simulink model "ModeStEnCtrlCaller"  (R2018b)
settings: Solver=FixedStepDiscrete  StartTime=0.0  StopTime=10.0  FixedStep=0.01  RelTol=1e-3
undefined symbols (not defined in the file): MdXX_DoneChk_Cal, ModeStEnCtrl4s_Cal, ModeStEnCtrl6s7s_Cal, ModeStEnCtrl6s7sPreCondition_Cal
settings Model: Creator=sn2xws  LastModifiedBy=sn2xws
settings DataIOCC: SaveFormat=StructureWithTime
settings OptimizationCC: DefaultParameterBehavior=Inlined  EnhancedBackFolding=on  PassReuseOutputArgsAs=Individual arguments  ZeroExternalMemoryAtStartup=off  ZeroInternalMemoryAtStartup=off  OptimizeBlockOrder=speed  DifferentSizesBufferReuse=on  OptimizationCustomize=off
settings DebuggingCC: ParameterTunabilityLossMsg=error
settings SFSimCC: MATLABDynamicMemAlloc=off
settings RTWCC: SystemTargetFile=autosar.tlc  GenCodeOnly=on  TemplateMakefile=ert_default_tmf  Description=AUTOSAR  GenerateReport=on  IncludeHyperlinkInReport=on  LaunchReport=on  GenerateTraceInfo=on  GenerateTraceReport=on  GenerateTraceReportSl=on  GenerateTraceReportSf=on  GenerateTraceReportEml=on  GenerateCodeMetricsReport=on
settings CodeAppCC: ForceParamTrailComments=on  IgnoreCustomStorageClasses=off  OperatorAnnotations=on  SimulinkDataObjDesc=on  SFDataObjDesc=on  InsertBlockDesc=on
settings STFCustomTargetCC: TargetLangStandard=C99 (ISO)  MultiwordLength=256  ParMdlRefBuildCompliant=on  CompOptLevelCompliant=on  IncludeMdlTerminateFcn=off  CombineOutputUpdateFcns=on  SuppressErrorStatus=on  ERTCustomFileBanners=on  SupportNonFinite=off  SupportComplex=off  SupportContinuousTime=off  SupportNonInlinedSFcns=off  RemoveResetFunc=on  MATLABClassNameForMDSCustomization=Simulink.SoftwareTarget.ERTCustomization  AutosarCompliant=on  UseToolchainInfoCompliant=on  LookupTableObjectStructAxisOrder=2,1,3,4,...  LUTObjectStructOrderEvenSpacing=Size,Table,Breakpoints  SystemTargetFile=autosar.tlc
settings ERTTargetCC: TargetLangStandard=C99 (ISO)  ConcurrentExecutionCompliant=off  IncludeMdlTerminateFcn=off  SuppressErrorStatus=on  SupportNonFinite=off  SupportComplex=off  ModelStepFunctionPrototypeControlCompliant=off  CPPClassGenCompliant=off  AutosarCompliant=on  LookupTableObjectStructAxisOrder=2,1,3,4,...  LUTObjectStructOrderEvenSpacing=Size,Table,Breakpoints  InlinedParameterPlacement=NonHierarchical  ERTCustomFileTemplate=example_file_process.tlc  ERTFilePackagingFormat=Compact

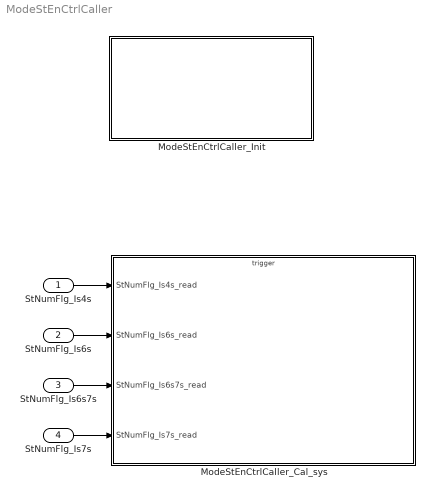
== system ModeStEnCtrlCaller ==
  StNumFlg_Is4s : Inport  OutDataTypeStr=boolean  PortDimensions=1
  StNumFlg_Is6s : Inport  Port=2  OutDataTypeStr=boolean  PortDimensions=1
  StNumFlg_Is6s7s : Inport  Port=3  OutDataTypeStr=boolean  PortDimensions=1
  StNumFlg_Is7s : Inport  Port=4  OutDataTypeStr=boolean  PortDimensions=1
  ModeStEnCtrlCaller_Cal_sys : Subsystem
  ModeStEnCtrlCaller_Init : Subsystem
  wires:
  StNumFlg_Is4s/1 -> ModeStEnCtrlCaller_Cal_sys/1(StNumFlg_Is4s_read)
  StNumFlg_Is6s/1 -> ModeStEnCtrlCaller_Cal_sys/2(StNumFlg_Is6s_read)
  StNumFlg_Is6s7s/1 -> ModeStEnCtrlCaller_Cal_sys/3(StNumFlg_Is6s7s_read)
  StNumFlg_Is7s/1 -> ModeStEnCtrlCaller_Cal_sys/4(StNumFlg_Is7s_read)

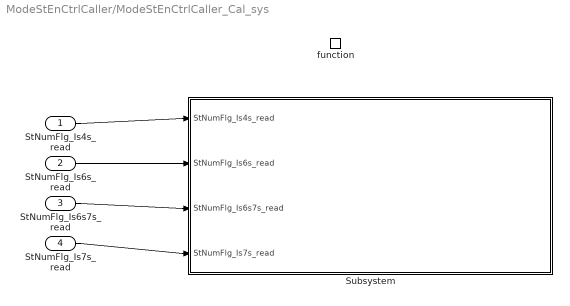
== system ModeStEnCtrlCaller/ModeStEnCtrlCaller_Cal_sys ==
  StNumFlg_Is4s_read : Inport
  StNumFlg_Is6s_read : Inport  Port=2
  StNumFlg_Is6s7s_read : Inport  Port=3
  StNumFlg_Is7s_read : Inport  Port=4
  function : TriggerPort  TriggerType=function-call  IsSimulinkFunction=on  FunctionName=ModeStEnCtrlCaller_Cal  VariantControl=(inherit)
  Subsystem : Subsystem
  wires:
  StNumFlg_Is4s_read/1 -> Subsystem/1(StNumFlg_Is4s_read)
  StNumFlg_Is6s_read/1 -> Subsystem/2(StNumFlg_Is6s_read)
  StNumFlg_Is6s7s_read/1 -> Subsystem/3(StNumFlg_Is6s7s_read)
  StNumFlg_Is7s_read/1 -> Subsystem/4(StNumFlg_Is7s_read)

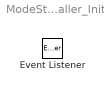
== system ModeStEnCtrlCaller/ModeStEnCtrlCaller_Init ==
  Event Listener : EventListener  EventName=reset

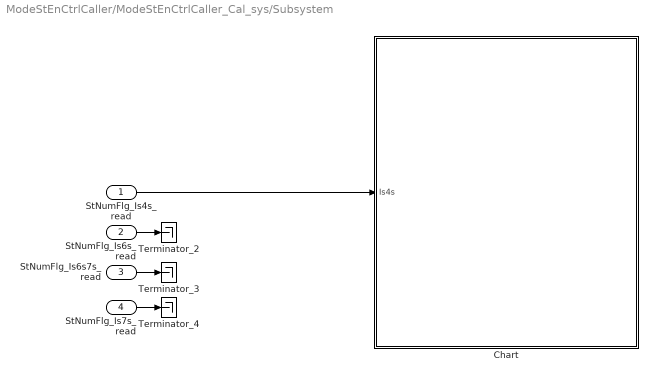
== system ModeStEnCtrlCaller/ModeStEnCtrlCaller_Cal_sys/Subsystem ==
  StNumFlg_Is4s_read : Inport
  StNumFlg_Is6s_read : Inport  Port=2
  StNumFlg_Is6s7s_read : Inport  Port=3
  StNumFlg_Is7s_read : Inport  Port=4
  Chart : Stateflow chart  TreatAsAtomicUnit=on
  Terminator_2 : Terminator
  Terminator_3 : Terminator
  Terminator_4 : Terminator
  wires:
  StNumFlg_Is7s_read/1 -> Terminator_4/1
  StNumFlg_Is4s_read/1 -> Chart/1(Is4s)
  StNumFlg_Is6s7s_read/1 -> Terminator_3/1
  StNumFlg_Is6s_read/1 -> Terminator_2/1

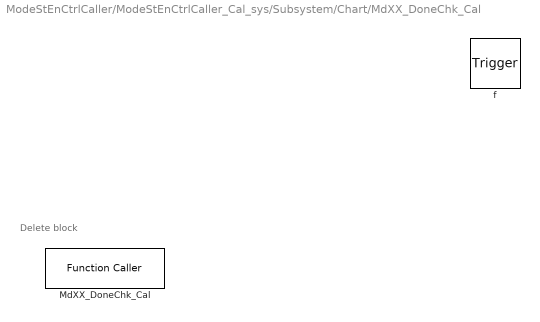
== system ModeStEnCtrlCaller/ModeStEnCtrlCaller_Cal_sys/Subsystem/Chart/MdXX_DoneChk_Cal ==
  note: Delete block
  f : TriggerPort  TriggerType=function-call  VariantControl=(inherit)
      settings: CopyFcn=Stateflow.SLINSF.SimulinkMan.removeBlockPreDeleteFcn  PreDeleteFcn=Stateflow.SLINSF.SimulinkMan.unsafePredeleteFcn
  MdXX_DoneChk_Cal : FunctionCaller  FunctionPrototype=MdXX_DoneChk_Cal()

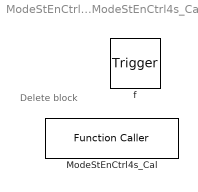
== system ModeStEnCtrlCaller/ModeStEnCtrlCaller_Cal_sys/Subsystem/Chart/ModeStEnCtrl4s_Cal ==
  note: Delete block
  f : TriggerPort  TriggerType=function-call  VariantControl=(inherit)
      settings: CopyFcn=Stateflow.SLINSF.SimulinkMan.removeBlockPreDeleteFcn  PreDeleteFcn=Stateflow.SLINSF.SimulinkMan.unsafePredeleteFcn
  ModeStEnCtrl4s_Cal : FunctionCaller  FunctionPrototype=ModeStEnCtrl4s_Cal()

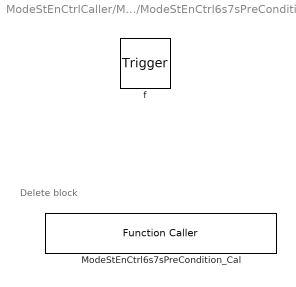
== system ModeStEnCtrlCaller/ModeStEnCtrlCaller_Cal_sys/Subsystem/Chart/ModeStEnCtrl6s7sPreCondition_Cal ==
  note: Delete block
  f : TriggerPort  TriggerType=function-call  VariantControl=(inherit)
      settings: CopyFcn=Stateflow.SLINSF.SimulinkMan.removeBlockPreDeleteFcn  PreDeleteFcn=Stateflow.SLINSF.SimulinkMan.unsafePredeleteFcn
  ModeStEnCtrl6s7sPreCondition_Cal : FunctionCaller  FunctionPrototype=ModeStEnCtrl6s7sPreCondition_Cal()

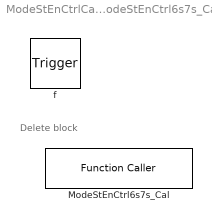
== system ModeStEnCtrlCaller/ModeStEnCtrlCaller_Cal_sys/Subsystem/Chart/ModeStEnCtrl6s7s_Cal ==
  note: Delete block
  f : TriggerPort  TriggerType=function-call  VariantControl=(inherit)
      settings: CopyFcn=Stateflow.SLINSF.SimulinkMan.removeBlockPreDeleteFcn  PreDeleteFcn=Stateflow.SLINSF.SimulinkMan.unsafePredeleteFcn
  ModeStEnCtrl6s7s_Cal : FunctionCaller  FunctionPrototype=ModeStEnCtrl6s7s_Cal()

== stateflow chart ModeStEnCtrlCaller/ModeStEnCtrlCaller_Cal_sys/Subsystem/Chart ==
  state ModeStEnCtrl4s_Cal [function]
  state ModeStEnCtrl6s7sPreCondition_Cal [function]
  state ModeStEnCtrl6s7s_Cal [function]
  state MdXX_DoneChk_Cal [function]
  (default) -> (junction 2)
  (junction 2) -> (junction 4) [order 1] : [Is4s]
  (junction 2) -> (junction 10) [order 2] : {
      | ModeStEnCtrl6s7sPreCondition_Cal();
      | ModeStEnCtrl6s7s_Cal();
      | }
  (junction 4) -> (junction 6) : {ModeStEnCtrl4s_Cal();}
  (junction 6) -> (junction 10)
  (junction 10) -> (junction 13) : {MdXX_DoneChk_Cal();}
  data: Is4s input
